simulink model "SOC_Estimation"  (R2020a)
settings: Solver=FixedStepDiscrete  StartTime=0.0  StopTime=10.0  FixedStep=0.05  RelTol=1e-3  EnableMultiTasking=on
InitFcn:
  | mbd_s32k_consistency_checks(bdroot(gcs));
values from neighbouring files (symbols this model uses):
  SOCInit = 0.75    [DD_SOC_Estimation.sldd]
  Ts = 0.1    [DD_SOC_Estimation.sldd]
undefined symbols (not defined in the file or in its folder): Battery, BMS_State_Enum, DiscIntNeverNeededParam, LQFP, Ns_Module, NumModules
libraries: simulink x6, sharedTrackingLibrary x2, mbd_s32k1xx_ec_toolbox x1
settings Model: DataDictionary=DD_SOC_Estimation.sldd  EnableAccessToBaseWorkspace=off  ExtModeTrigDuration=5  Creator=cpatel  LastModifiedBy=RolandoA
settings SolverCC: AutoInsertRateTranBlk=on
settings DataIOCC: ExternalInput=off  InitialState=off  SaveOutput=off  SignalLogging=off  SaveTime=off
settings OptimizationCC: DefaultParameterBehavior=Inlined  EnhancedBackFolding=on  PassReuseOutputArgsAs=Individual arguments  ZeroExternalMemoryAtStartup=off  ZeroInternalMemoryAtStartup=off  OptimizeBlockOrder=speed  DifferentSizesBufferReuse=on  OptimizationCustomize=off  EfficientTunableParamExpr=on
settings DebuggingCC: UnderspecifiedInitializationDetection=Classic  MergeDetectMultiDrivingBlocksExec=none  InheritedTsInSrcMsg=none  SingleTaskRateTransMsg=error  ParameterTunabilityLossMsg=error  UnconnectedInputMsg=error  UnconnectedOutputMsg=error  UnconnectedLineMsg=error  UnknownTsInhSupMsg=error
settings HardwareCC: ProdBitPerPointer=32  ProdBitPerSizeT=32  ProdBitPerPtrDiffT=32  ProdLargestAtomicInteger=Long  ProdLargestAtomicFloat=Double  ProdWordSize=32  ProdHWDeviceType=ARM Compatible->ARM Cortex
settings ModelReferenceCC: ModelReferenceNumInstancesAllowed=Single  PropagateSignalLabelsOutOfModel=off
settings SFSimCC: MATLABDynamicMemAlloc=off
settings RTWCC: Description=Model Based Design Toolbox S32K1xx Code Generation Target  SystemTargetFile=mbd_s32k.tlc  MakeCommand=mbd_s32k_make_rtw COPY_MDLREF_INCLUDES=0  TemplateMakefile=mbd_s32k.tmf  GenerateReport=on  IncludeHyperlinkInReport=on  LaunchReport=on  GenerateTraceInfo=on  GenerateTraceReport=on  GenerateTraceReportSl=on  GenerateTraceReportSf=on  GenerateTraceReportEml=on
settings CodeAppCC: ForceParamTrailComments=on  IgnoreCustomStorageClasses=off  OperatorAnnotations=on  SimulinkDataObjDesc=on  SFDataObjDesc=on  InsertBlockDesc=on
settings STFCustomTargetCC: TargetLangStandard=C99 (ISO)  MultiwordLength=256  CombineOutputUpdateFcns=on  ERTCustomFileBanners=on  SupportContinuousTime=off  SupportNonInlinedSFcns=off  RemoveResetFunc=on  MATLABClassNameForMDSCustomization=Simulink.SoftwareTarget.ERTCustomization  SystemTargetFile=mbd_s32k.tlc
settings ERTTargetCC: TargetLangStandard=C99 (ISO)  ParMdlRefBuildCompliant=off  CompOptLevelCompliant=off  ConcurrentExecutionCompliant=off  ModelStepFunctionPrototypeControlCompliant=off  CPPClassGenCompliant=off  UseToolchainInfoCompliant=off  InlinedParameterPlacement=NonHierarchical  ERTSrcFileBannerTemplate=mbd_ert_code_template.cgt  ERTHdrFileBannerTemplate=mbd_ert_code_template.cgt  ERTDataSrcFileTemplate=mbd_ert_code_template.cgt  ERTDataHdrFileTemplate=mbd_ert_code_template.cgt  ERTCustomFileTemplate=example_file_process.tlc

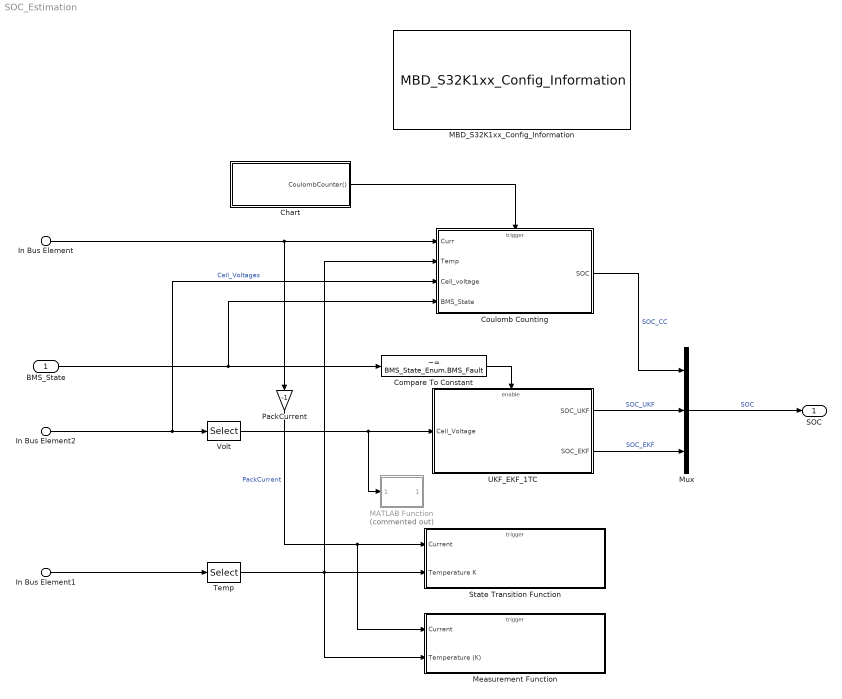
== system SOC_Estimation ==
  BMS_State : Inport  OutDataTypeStr=Enum: BMS_State_Enum
  In Bus Element2 : Inport  Port=2  PortName=BMS_Input  Element=Cell_Voltages
  In Bus Element : Inport  Port=2  PortName=BMS_Input  Element=Pack_Current
  In Bus Element1 : Inport  Port=2  PortName=BMS_Input  Element=Cell_Temperatures
  Chart : Stateflow chart  TreatAsAtomicUnit=on
  Compare To Constant : simulink/Logic and Bit Operations/Compare To Constant  relop=~=  const=BMS_State_Enum.BMS_Fault  OutDataTypeStr=boolean
  Coulomb Counting : Subsystem  VariantControl=SocAlgo==1
  MATLAB Function : MATLAB Function  Commented=on  TreatAsAtomicUnit=on
  MBD_S32K1xx_Config_Information : mbd_s32k1xx_ec_toolbox/MBD_S32K1xx_Config_Information  mbdt_ver=0  disp_str=|  config_params=[]  mcu_target_name=S32K144  mcu_target_package=100-LQFP  mcu_target_sram_size=64KB  mcu_system_clock_freq=80  mcu_xtal_freq=External 8  mcu_steptick_timer=LPIT Channel 0  mcu_steptick_prio=15  ds_import_enable=on  target_compiler=GCC  target_memory=FLASH  gcc_target_compile_opts=-mthumb -mfloat-abi=hard -mfpu=fpv4-sp-d16 -O1 -g -gstrict-dwarf  gcc_target_assemble_opts=-mthumb -mfloat-abi=hard -mfpu=fpv4-sp-d16 -g  gcc_target_link_opts=-mthumb -mfloat-abi=hard -mfpu=fpv4-sp-d16  gcc_target_default_lcf=on  gcc_target_user_lcf=S32K148_192_flash.ld  ghs_target_compile_opts=-cpu=cortexm4f -thumb -fpu=vfpv4_d16 -fsingle -Ogeneral -Wundef -Wimplicit-int -Wshadow -Wtrigraphs --no_commons --gnu_asm -gnu99 -gdwarf-2 -G  ghs_target_assemble_opts=-cpu=cortexm4f -fpu=vfpv4_d16  ghs_target_link_opts=-cpu=cortexm4f -thumb -fpu=vfpv4_d16  ghs_target_default_lcf=on  ghs_target_user_lcf=S32K148_192_flash.ld  iar_target_compile_opts=--cpu=Cortex-M4F --thumb --fpu=VFPv4_sp -Ol -e --debug --dlib_config normal  iar_target_assemble_opts=--cpu Cortex-M4F --thumb --fpu VFPv4_sp  iar_target_link_opts=--no_exceptions --vfe --inline  iar_target_default_lcf=on  iar_target_user_lcf=S32K148_192_flash.icf  pil_download_enable=off  rbl_download_enable=on  rbl_start_delay=5000  rbl_download_interface=OpenSDA  rbl_restart_request=off  rbl_com_port=Custom  rbl_com_port_custom=COM1  pil_download_rate=57600  pil_opensda_drive=Custom  pil_opensda_drive_custom=D  pil_uart_instance=1  pil_uart_rx=PTC6: [LPUART1_RX | Receive]  pil_uart_tx=PTC7: [LPUART1_TX | Transmit]  FTM_PWM_PcrCheckEnDis=on  FTM_Input_Edge_Inputs_PcrCheckEnDis=on  FTM_Dual_Edge_Inputs_PcrCheckEnDis=on  FTM_Quadrature_Inputs_PcrCheckEnDis=on  FTM_Hall_Sensor_Inputs_PcrCheckEnDis=on  LPTMR_PcrCheckEnDis=on  PIT_PcrCheckEnDis=on  RTC_PcrCheckEnDis=on  FlexCAN_PcrCheckEnDis=on  LIN_PcrCheckEnDis=on  FlexIO_PcrCheckEnDis=on  LPI2C_PcrCheckEnDis=on  LPSPI_PcrCheckEnDis=on  LPUART_PcrCheckEnDis=on  CMP_PcrCheckEnDis=on  GPIO_OutputPcrCheckEnDis=on  GPIO_InputPcrCheckEnDis=on  SBC_PcrCheckEnDis=on  BMS_PcrCheckEnDis=on  AMMCLIB_PcrCheckEnDis=on  FM_PcrCheckEnDis=on  Profile_PcrCheckEnDis=on  ConfigParams_PcrCheckEnDis=on  ModelRef_PcrCheckEnDis=on  PDB0_PcrCheckEnDis=on  CSEc_PcrCheckEnDis=on  eDMA_PcrCheckEnDis=on  FLASH_PcrCheckEnDis=on  ADC_PcrCheckEnDis=on  WDOG_PcrCheckEnDis=on
      | Target : S32K144-64KB_SRAM
      | Package : 100-pin
      | System clock : 80 MHz
      | XTAL clock : External 8 MHz
      | Compiler : IAR
      | Target Type : FLASH
      | Download Code after build : off
      | Step Tick Interrupt Priority : 15
  Measurement Function : Subsystem  TreatAsAtomicUnit=on
  Mux : Mux  Inputs=3
  PackCurrent : Gain  Gain=-1
  State Transition Function : Subsystem  TreatAsAtomicUnit=on
  Temp : Selector  InputPortWidth=Ns_Module*NumModules - 6  IndexOptions=Index vector (dialog)  Indices=[1]  OutputSizes=1
  UKF_EKF_1TC : Subsystem  VariantControl=CellType==1
  Volt : Selector  InputPortWidth=Ns_Module*NumModules  IndexOptions=Index vector (dialog)  Indices=[1]  OutputSizes=1
  SOC : Outport  OutDataTypeStr=single  VectorParamsAs1DForOutWhenUnconnected=off
  wires:
  In Bus Element2/1 -> Coulomb Counting/3(Cell_voltage), Volt/1  "Cell_Voltages"
  In Bus Element1/1 -> Temp/1
  Mux/1 -> SOC/1  "SOC"
  In Bus Element/1 -> Coulomb Counting/1(Curr), PackCurrent/1
  BMS_State/1 -> Coulomb Counting/4(BMS_State), Compare To Constant/1
  Compare To Constant/1 -> UKF_EKF_1TC/Enable
  PackCurrent/1 -> State Transition Function/1(Current), Measurement Function/1(Current)  "PackCurrent"
  Temp/1 -> Measurement Function/2(Temperature (K)), Coulomb Counting/2(Temp), State Transition Function/2(Temperature K)
  Volt/1 -> UKF_EKF_1TC/1(Cell_Voltage), MATLAB Function/1(meas)
  UKF_EKF_1TC/2(SOC_EKF) -> Mux/3  "SOC_EKF"
  UKF_EKF_1TC/1(SOC_UKF) -> Mux/2  "SOC_UKF"
  Chart/1(CoulombCounter()) -> Coulomb Counting/Trigger
  Coulomb Counting/1(SOC) -> Mux/1  "SOC_CC"

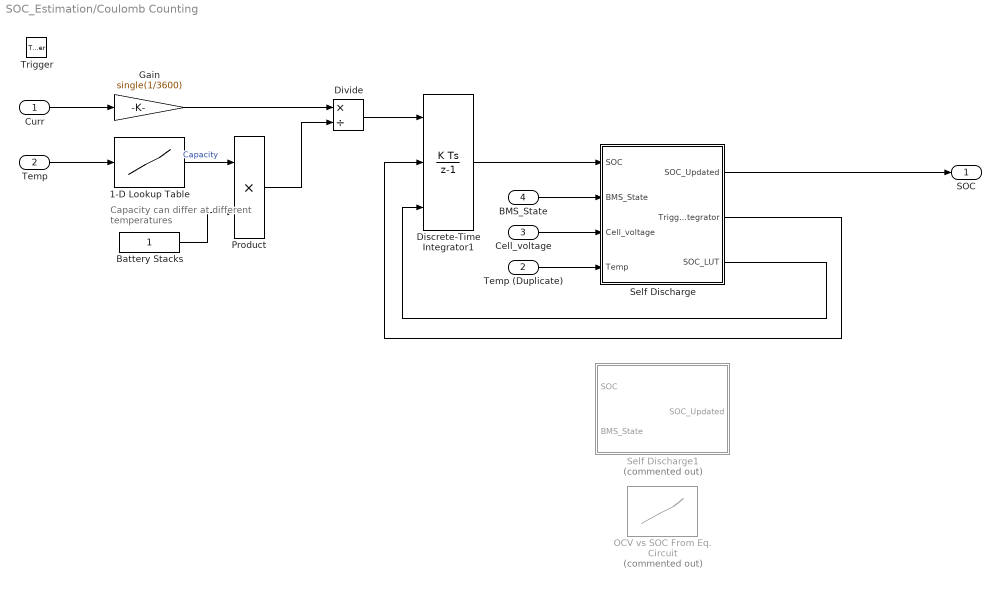
== system SOC_Estimation/Coulomb Counting ==
  note: Capacity can differ at different temperatures
  Curr : Inport
  Temp : Inport  Port=2
  Cell_voltage : Inport  Port=3
  BMS_State : Inport  Port=4
  Trigger : TriggerPort  TriggerType=function-call  VariantControl=Variant  PortDimensions=1
  1-D Lookup Table : Lookup_n-D  NumberOfTableDimensions=1  BreakpointsForDimension1=single(Battery.Temperature_LUT)  Table=single(Battery.Capacity_LUT)  InternalRulePriority=Speed  RndMeth=Simplest  InputSameDT=on
  Battery Stacks : Constant  OutDataTypeStr=single
  Discrete-Time Integrator1 : DiscreteIntegrator  ExternalReset=rising  InitialConditionSource=external  InitialCondition=single(SOCInit+0.05)  SampleTime=-1  LimitOutput=on  UpperSaturationLimit=1  LowerSaturationLimit=0  ICPrevOutput=DiscIntNeverNeededParam  ICPrevScaledInput=DiscIntNeverNeededParam
  Divide : Product  Inputs=*/
  Gain : Gain  Gain=single(1/3600)
  OCV vs SOC From Eq. Circuit : Lookup_n-D  Commented=on  NumberOfTableDimensions=1  BreakpointsForDimension1=single(Battery.Em_LUT1D)  Table=single(Battery.SOC_LUT)  InternalRulePriority=Speed  RndMeth=Simplest  InputSameDT=on
  Product : Product
  Self Discharge : Subsystem
  Self Discharge1 : Subsystem  Commented=on
  Temp (Duplicate) : InportShadow  Port=2
  SOC : Outport  VectorParamsAs1DForOutWhenUnconnected=off
  wires:
  Curr/1 -> Gain/1
  Gain/1 -> Divide/1
  Temp/1 -> 1-D Lookup Table/1
  1-D Lookup Table/1 -> Product/1  "Capacity"
  Product/1 -> Divide/2
  Battery Stacks/1 -> Product/2
  Self Discharge/1(SOC_Updated) -> SOC/1
  Self Discharge/2(Trigger_integrator) -> Discrete-Time Integrator1/2
  Self Discharge/3(SOC_LUT) -> Discrete-Time Integrator1/3
  Discrete-Time Integrator1/1 -> Self Discharge/1(SOC)
  Divide/1 -> Discrete-Time Integrator1/1
  BMS_State/1 -> Self Discharge/2(BMS_State)
  Cell_voltage/1 -> Self Discharge/3(Cell_voltage)
  Temp (Duplicate)/1 -> Self Discharge/4(Temp)

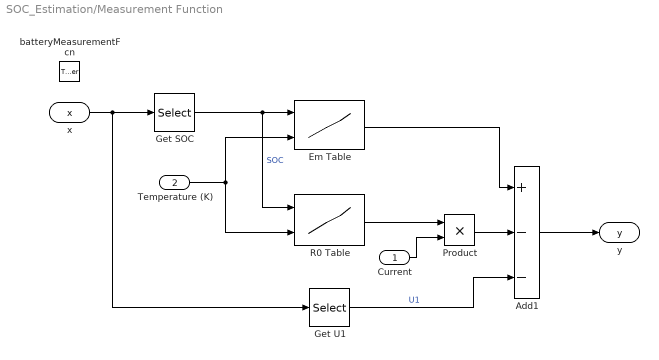
== system SOC_Estimation/Measurement Function ==
  Current : Inport
  Temperature (K) : Inport  Port=2
  batteryMeasurementFcn : TriggerPort  TriggerType=function-call  IsSimulinkFunction=on  FunctionName=batteryMeasurementFcn  VariantControl=Variant
  Add1 : Sum  Inputs=+--
  Em Table : Lookup_n-D  BreakpointsForDimension1=Battery.SOC_LUT  BreakpointsForDimension2=Battery.Temperature_LUT  BeginIndexSearchUsingPreviousIndexResult=on  Table=Battery.Em_LUT  ExtrapMethod=Clip  InternalRulePriority=Speed  RndMeth=Simplest  InputSameDT=on
  Get SOC : Selector  InputPortWidth=2  IndexOptions=Index vector (dialog)  Indices=[1]  OutputSizes=1
  Get U1 : Selector  InputPortWidth=2  IndexOptions=Index vector (dialog)  Indices=2  OutputSizes=1
  Product : Product
  R0 Table : Lookup_n-D  BreakpointsForDimension1=Battery.SOC_LUT  BreakpointsForDimension2=Battery.Temperature_LUT  BeginIndexSearchUsingPreviousIndexResult=on  Table=Battery.R0_LUT  ExtrapMethod=Clip  InternalRulePriority=Speed  RndMeth=Simplest  InputSameDT=on
  x : ArgIn  DisableCoverage=on  OutDataTypeStr=single  PortDimensions=2  ArgumentName=x
  y : ArgOut  DisableCoverage=on  OutDataTypeStr=single  ArgumentName=y
  wires:
  Get U1/1 -> Add1/3  "U1"
  Product/1 -> Add1/2
  Current/1 -> Product/2
  R0 Table/1 -> Product/1
  Temperature (K)/1 -> Em Table/2, R0 Table/2
  Add1/1 -> y/1
  Em Table/1 -> Add1/1
  Get SOC/1 -> Em Table/1, R0 Table/1  "SOC"
  x/1 -> Get SOC/1, Get U1/1

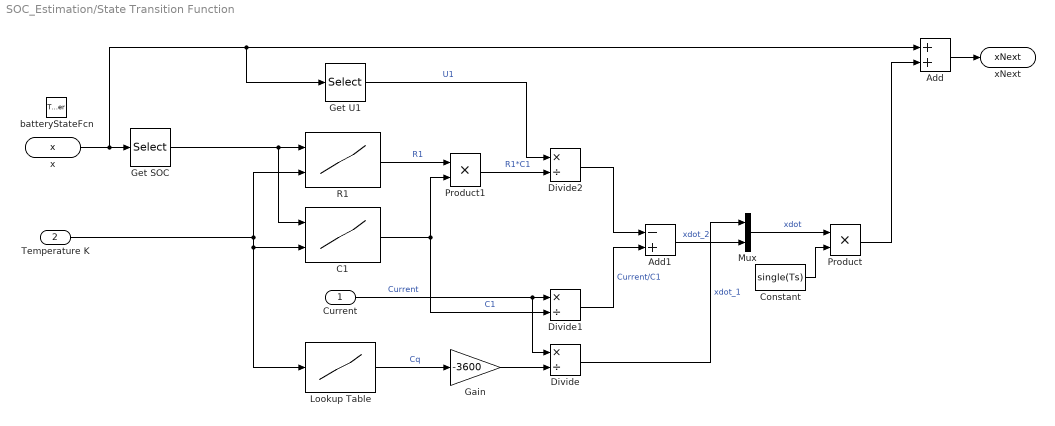
== system SOC_Estimation/State Transition Function ==
  Current : Inport
  Temperature K : Inport  Port=2
  batteryStateFcn : TriggerPort  TriggerType=function-call  IsSimulinkFunction=on  FunctionName=batteryStateFcn  VariantControl=Variant
  Add : Sum
  Add1 : Sum  Inputs=-+
  C1 : Lookup_n-D  BreakpointsForDimension1=Battery.SOC_LUT  BreakpointsForDimension2=Battery.Temperature_LUT  BeginIndexSearchUsingPreviousIndexResult=on  Table=Battery.C1_LUT  ExtrapMethod=Clip  InternalRulePriority=Speed  RndMeth=Simplest  InputSameDT=on
  Constant : Constant  Value=single(Ts)  OutDataTypeStr=single
  Divide : Product  Inputs=*/
  Divide1 : Product  Inputs=*/
  Divide2 : Product  Inputs=*/
  Gain : Gain  Gain=-3600
  Get SOC : Selector  InputPortWidth=2  IndexOptions=Index vector (dialog)  Indices=1  OutputSizes=1
  Get U1 : Selector  InputPortWidth=2  IndexOptions=Index vector (dialog)  Indices=2  OutputSizes=1
  Lookup Table : Lookup_n-D  NumberOfTableDimensions=1  BreakpointsForDimension1=Battery.Temperature_LUT  BeginIndexSearchUsingPreviousIndexResult=on  Table=Battery.Capacity_LUT  InternalRulePriority=Speed  RndMeth=Simplest  InputSameDT=on
  Mux : Mux  Inputs=2
  Product : Product  OutDataTypeStr=single
  Product1 : Product
  R1 : Lookup_n-D  BreakpointsForDimension1=Battery.SOC_LUT  BreakpointsForDimension2=Battery.Temperature_LUT  BeginIndexSearchUsingPreviousIndexResult=on  Table=Battery.R1_LUT  ExtrapMethod=Clip  InternalRulePriority=Speed  RndMeth=Simplest  InputSameDT=on
  x : ArgIn  DisableCoverage=on  OutDataTypeStr=single  PortDimensions=2  ArgumentName=x
  xNext : ArgOut  DisableCoverage=on  OutDataTypeStr=single  PortDimensions=2  ArgumentName=xNext
  wires:
  Lookup Table/1 -> Gain/1  "Cq"
  Product/1 -> Add/2
  Constant/1 -> Product/2
  Current/1 -> Divide1/1, Divide/1  "Current"
  Get SOC/1 -> C1/1, R1/1
  Temperature K/1 -> Lookup Table/1, C1/2, R1/2
  Add/1 -> xNext/1
  x/1 -> Add/1, Get U1/1, Get SOC/1
  Gain/1 -> Divide/2
  Divide/1 -> Mux/1  "xdot_1"
  Get U1/1 -> Divide2/1  "U1"
  Product1/1 -> Divide2/2  "R1*C1"
  R1/1 -> Product1/1  "R1"
  C1/1 -> Product1/2, Divide1/2  "C1"
  Divide1/1 -> Add1/2  "Current/C1"
  Divide2/1 -> Add1/1
  Add1/1 -> Mux/2  "xdot_2"
  Mux/1 -> Product/1  "xdot"

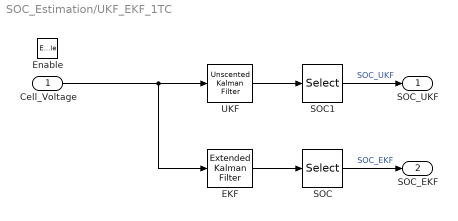
== system SOC_Estimation/UKF_EKF_1TC ==
  Cell_Voltage : Inport
  Enable : EnablePort
  EKF : sharedTrackingLibrary/Extended Kalman Filter  StateTransitionFcn=batteryStateFcn  HasStateTransitionJacobianFcn=off  HasAdditiveProcessNoise=Additive  ProcessNoise=1e-10*eye(2)  HasTimeVaryingProcessNoise=off  HasStateTransitionFcnExtraArgument=0  InitialState=[single(SOCInit+0.05); 0;]  InitialStateCovariance=[1e-5 1]  MeasurementFcn1=batteryMeasurementFcn  HasMeasurementJacobianFcn1=off  HasMeasurementEnablePort1=off  HasAdditiveMeasurementNoise1=Additive  MeasurementNoise1=1e-1  HasTimeVaryingMeasurementNoise1=off  HasMeasurementFcnExtraArgument1=0  MeasurementFcn2=myMeasurementFcn  HasMeasurementJacobianFcn2=off  HasMeasurementEnablePort2=off  HasAdditiveMeasurementNoise2=Additive  MeasurementNoise2=1  HasTimeVaryingMeasurementNoise2=off  HasMeasurementFcnExtraArgument2=0  MeasurementFcn3=myMeasurementFcn  HasMeasurementJacobianFcn3=off  HasMeasurementEnablePort3=off  HasAdditiveMeasurementNoise3=Additive  MeasurementNoise3=1  HasTimeVaryingMeasurementNoise3=off  HasMeasurementFcnExtraArgument3=0  MeasurementFcn4=myMeasurementFcn  HasMeasurementJacobianFcn4=off  HasMeasurementEnablePort4=off  HasAdditiveMeasurementNoise4=Additive  MeasurementNoise4=1  HasTimeVaryingMeasurementNoise4=off  HasMeasurementFcnExtraArgument4=0  MeasurementFcn5=myMeasurementFcn  HasMeasurementJacobianFcn5=off  HasMeasurementEnablePort5=off  HasAdditiveMeasurementNoise5=Additive  MeasurementNoise5=1  HasTimeVaryingMeasurementNoise5=off  HasMeasurementFcnExtraArgument5=0  EnableMultirate=off  StateTransitionFcnSampleTime=1  MeasurementFcn1SampleTime=1  MeasurementFcn2SampleTime=1  MeasurementFcn3SampleTime=1  MeasurementFcn4SampleTime=1  MeasurementFcn5SampleTime=1  UseCurrentEstimator=on  OutputStateCovariance=off  DataType=single  SampleTime=Ts  NumberOfMeasurements=1
      settings: SourceProductBaseCode=CT,DR,TF,ID,NV,AR,RO,VE
  SOC : Selector  InputPortWidth=2  IndexOptions=Index vector (dialog)  Indices=1  OutputSizes=1
  SOC1 : Selector  InputPortWidth=2  IndexOptions=Index vector (dialog)  Indices=1  OutputSizes=1
  UKF : sharedTrackingLibrary/Unscented Kalman Filter  StateTransitionFcn=batteryStateFcn  HasAdditiveProcessNoise=Additive  ProcessNoise=1e-10*eye(2)  HasTimeVaryingProcessNoise=off  HasStateTransitionFcnExtraArgument=0  InitialState=[single(SOCInit+0.05); 0;]  InitialStateCovariance=[1e-5 1]  Alpha=1  Beta=2  Kappa=1  MeasurementFcn1=batteryMeasurementFcn  HasMeasurementEnablePort1=off  HasAdditiveMeasurementNoise1=Additive  MeasurementNoise1=0.1  HasTimeVaryingMeasurementNoise1=off  HasMeasurementFcnExtraArgument1=0  MeasurementFcn2=myMeasurementFcn  HasMeasurementEnablePort2=off  HasAdditiveMeasurementNoise2=Additive  MeasurementNoise2=1  HasTimeVaryingMeasurementNoise2=off  HasMeasurementFcnExtraArgument2=0  MeasurementFcn3=myMeasurementFcn  HasMeasurementEnablePort3=off  HasAdditiveMeasurementNoise3=Additive  MeasurementNoise3=1  HasTimeVaryingMeasurementNoise3=off  HasMeasurementFcnExtraArgument3=0  MeasurementFcn4=myMeasurementFcn  HasMeasurementEnablePort4=off  HasAdditiveMeasurementNoise4=Additive  MeasurementNoise4=1  HasTimeVaryingMeasurementNoise4=off  HasMeasurementFcnExtraArgument4=0  MeasurementFcn5=myMeasurementFcn  HasMeasurementEnablePort5=off  HasAdditiveMeasurementNoise5=Additive  MeasurementNoise5=1  HasTimeVaryingMeasurementNoise5=off  HasMeasurementFcnExtraArgument5=0  EnableMultirate=off  StateTransitionFcnSampleTime=-1  MeasurementFcn1SampleTime=-1  MeasurementFcn2SampleTime=-1  MeasurementFcn3SampleTime=-1  MeasurementFcn4SampleTime=-1  MeasurementFcn5SampleTime=-1  UseCurrentEstimator=on  OutputStateCovariance=off  DataType=single  SampleTime=Ts  NumberOfMeasurements=1
      settings: SourceProductBaseCode=CT,DR,TF,ID,NV,AR,RO,VE
  SOC_UKF : Outport  VectorParamsAs1DForOutWhenUnconnected=off
  SOC_EKF : Outport  Port=2  VectorParamsAs1DForOutWhenUnconnected=off
  wires:
  UKF/1 -> SOC1/1
  Cell_Voltage/1 -> UKF/1, EKF/1
  SOC1/1 -> SOC_UKF/1  "SOC_UKF"
  EKF/1 -> SOC/1
  SOC/1 -> SOC_EKF/1  "SOC_EKF"

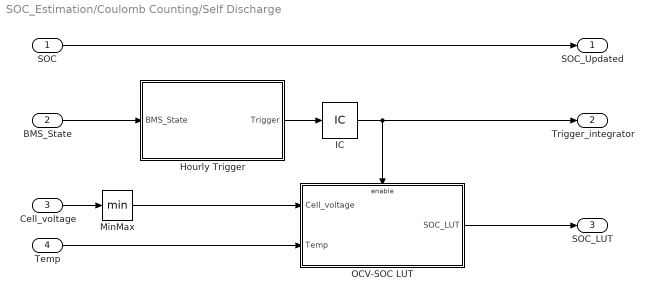
== system SOC_Estimation/Coulomb Counting/Self Discharge ==
  SOC : Inport
  BMS_State : Inport  Port=2
  Cell_voltage : Inport  Port=3
  Temp : Inport  Port=4
  Hourly Trigger : Subsystem
  IC : InitialCondition
  MinMax : MinMax
  OCV-SOC LUT : Subsystem
  SOC_Updated : Outport
  Trigger_integrator : Outport  Port=2
  SOC_LUT : Outport  Port=3
  wires:
  Hourly Trigger/1(Trigger) -> IC/1
  BMS_State/1 -> Hourly Trigger/1(BMS_State)
  SOC/1 -> SOC_Updated/1
  Cell_voltage/1 -> MinMax/1
  OCV-SOC LUT/1(SOC_LUT) -> SOC_LUT/1
  IC/1 -> Trigger_integrator/1, OCV-SOC LUT/Enable
  MinMax/1 -> OCV-SOC LUT/1(Cell_voltage)
  Temp/1 -> OCV-SOC LUT/2(Temp)

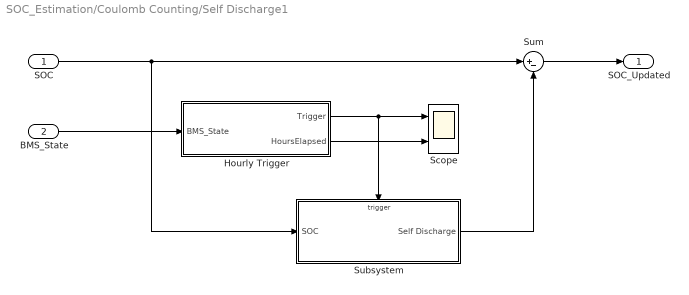
== system SOC_Estimation/Coulomb Counting/Self Discharge1 ==
  SOC : Inport
  BMS_State : Inport  Port=2
  Hourly Trigger : Subsystem
  Scope : Scope  NumInputPorts=2
  Subsystem : Subsystem
  Sum : Sum  Inputs=|+-
  SOC_Updated : Outport
  wires:
  SOC/1 -> Subsystem/1(SOC), Sum/1
  Sum/1 -> SOC_Updated/1
  Subsystem/1(Self Discharge) -> Sum/2
  BMS_State/1 -> Hourly Trigger/1(BMS_State)
  Hourly Trigger/1(Trigger) -> Scope/1, Subsystem/Trigger
  Hourly Trigger/2(HoursElapsed) -> Scope/2

== system SOC_Estimation/Coulomb Counting/Self Discharge/Hourly Trigger ==
  BMS_State : Inport
  1hr Trigger : Subsystem
  Compare To Constant1 : simulink/Logic and Bit Operations/Compare To Constant  relop===  const=BMS_State_Enum.BMS_Standby  OutDataTypeStr=boolean
  Trigger : Outport
  wires:
  BMS_State/1 -> Compare To Constant1/1
  Compare To Constant1/1 -> 1hr Trigger/Enable
  1hr Trigger/1(Trigger) -> Trigger/1

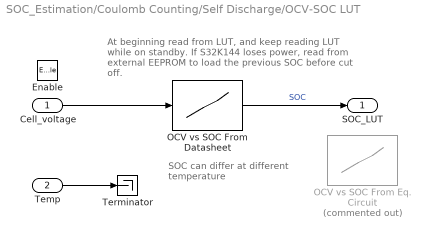
== system SOC_Estimation/Coulomb Counting/Self Discharge/OCV-SOC LUT ==
  note: SOC can differ at different temperature
  note: At beginning read from LUT, and keep reading LUT while on standby. If S32K144 loses power, read from external EEPROM to load the previous SOC before cut off.
  Cell_voltage : Inport
  Temp : Inport  Port=2
  Enable : EnablePort
  OCV vs SOC From Datasheet : Lookup_n-D  NumberOfTableDimensions=1  BreakpointsForDimension1=single(Battery.OCVLUT_DS)  Table=single(Battery.SOCLUT_DS)  InternalRulePriority=Speed  RndMeth=Simplest  InputSameDT=on
  OCV vs SOC From Eq. Circuit : Lookup_n-D  Commented=on  NumberOfTableDimensions=1  BreakpointsForDimension1=single(Battery.Em_LUT1D)  Table=single(Battery.SOC_LUT)  InternalRulePriority=Speed  RndMeth=Simplest  InputSameDT=on
  Terminator : Terminator
  SOC_LUT : Outport
  wires:
  OCV vs SOC From Datasheet/1 -> SOC_LUT/1  "SOC"
  Cell_voltage/1 -> OCV vs SOC From Datasheet/1
  Temp/1 -> Terminator/1

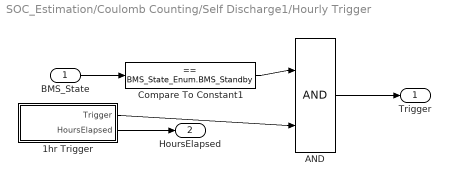
== system SOC_Estimation/Coulomb Counting/Self Discharge1/Hourly Trigger ==
  BMS_State : Inport
  1hr Trigger : Subsystem
  AND : Logic  IconShape=distinctive  AllPortsSameDT=off  OutDataTypeStr=boolean
  Compare To Constant1 : simulink/Logic and Bit Operations/Compare To Constant  relop===  const=BMS_State_Enum.BMS_Standby  OutDataTypeStr=boolean
  Trigger : Outport
  HoursElapsed : Outport  Port=2
  wires:
  BMS_State/1 -> Compare To Constant1/1
  AND/1 -> Trigger/1
  1hr Trigger/1(Trigger) -> AND/2
  1hr Trigger/2(HoursElapsed) -> HoursElapsed/1
  Compare To Constant1/1 -> AND/1

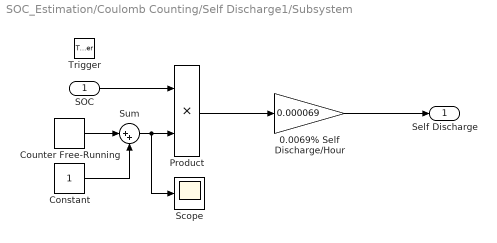
== system SOC_Estimation/Coulomb Counting/Self Discharge1/Subsystem ==
  SOC : Inport
  Trigger : TriggerPort  VariantControl=Variant  PortDimensions=1
  0.0069% Self Discharge/Hour : Gain  Gain=0.000069
  Constant : Constant
  Counter Free-Running : simulink/Sources/Counter Free-Running  NumBits=64  tsamp=-1
  Product : Product
  Scope : Scope
  Sum : Sum  Inputs=|++
  Self Discharge : Outport
  wires:
  Product/1 -> 0.0069% Self Discharge/Hour/1
  0.0069% Self Discharge/Hour/1 -> Self Discharge/1
  SOC/1 -> Product/1
  Sum/1 -> Scope/1, Product/2
  Counter Free-Running/1 -> Sum/1
  Constant/1 -> Sum/2

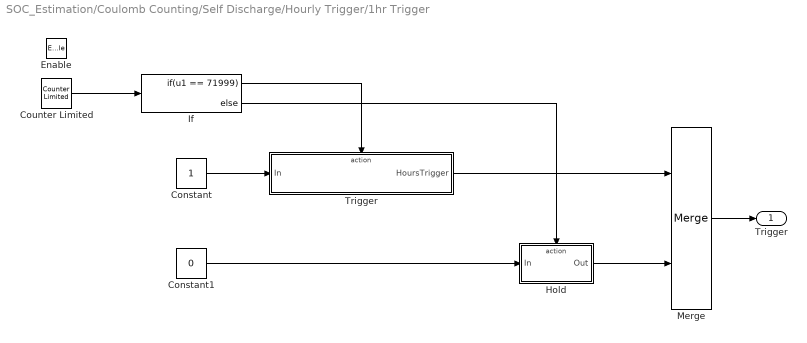
== system SOC_Estimation/Coulomb Counting/Self Discharge/Hourly Trigger/1hr Trigger ==
  Enable : EnablePort  StatesWhenEnabling=reset
  " Trigger" : Subsystem  TreatAsAtomicUnit=on
  Constant : Constant  OutDataTypeStr=uint16
  Constant1 : Constant  Value=0  OutDataTypeStr=uint16
  Counter Limited : simulink/Sources/Counter Limited  uplimit=71999  tsamp=-1
  Hold : Subsystem  TreatAsAtomicUnit=on
  If : If  IfExpression=u1 == 71999
  Merge : Merge
  Trigger : Outport  OutputWhenDisabled=reset  InitialOutput=0
  wires:
  " Trigger"/1(HoursTrigger) -> Merge/1
  If/1 -> " Trigger"/Action
  If/2 -> Hold/Action
  Merge/1 -> Trigger/1
  Constant1/1 -> Hold/1(In)
  Counter Limited/1 -> If/1
  Hold/1(Out) -> Merge/2
  Constant/1 -> " Trigger"/1(In)

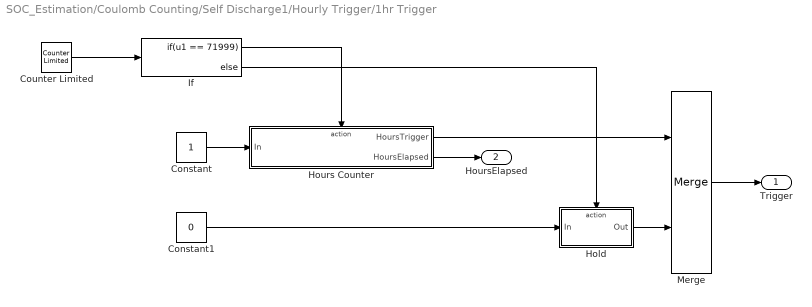
== system SOC_Estimation/Coulomb Counting/Self Discharge1/Hourly Trigger/1hr Trigger ==
  Constant : Constant  OutDataTypeStr=uint16
  Constant1 : Constant  Value=0  OutDataTypeStr=uint16
  Counter Limited : simulink/Sources/Counter Limited  uplimit=71999  tsamp=-1
  Hold : Subsystem  TreatAsAtomicUnit=on
  Hours Counter : Subsystem  TreatAsAtomicUnit=on
  If : If  IfExpression=u1 == 71999
  Merge : Merge
  Trigger : Outport
  HoursElapsed : Outport  Port=2
  wires:
  Constant/1 -> Hours Counter/1(In)
  Hold/1(Out) -> Merge/2
  Counter Limited/1 -> If/1
  Constant1/1 -> Hold/1(In)
  Merge/1 -> Trigger/1
  If/2 -> Hold/Action
  If/1 -> Hours Counter/Action
  Hours Counter/2(HoursElapsed) -> HoursElapsed/1
  Hours Counter/1(HoursTrigger) -> Merge/1

== system SOC_Estimation/Coulomb Counting/Self Discharge/Hourly Trigger/1hr Trigger/ Trigger ==
  In : Inport
  Action Port : ActionPort  ActionPortLabel=if(u1 == 71999)
  HoursTrigger : Outport  InitialOutput=0
  wires:
  In/1 -> HoursTrigger/1

== system SOC_Estimation/Coulomb Counting/Self Discharge/Hourly Trigger/1hr Trigger/Hold ==
  In : Inport
  Action Port : ActionPort  ActionPortLabel=else
  Out : Outport
  wires:
  In/1 -> Out/1

== system SOC_Estimation/Coulomb Counting/Self Discharge1/Hourly Trigger/1hr Trigger/Hold ==
  In : Inport
  Action Port : ActionPort
  Out : Outport
  wires:
  In/1 -> Out/1

== system SOC_Estimation/Coulomb Counting/Self Discharge1/Hourly Trigger/1hr Trigger/Hours Counter ==
  In : Inport
  Action Port : ActionPort
  Sum : Sum  Inputs=|++
  Unit Delay : UnitDelay  SampleTime=-1  HasFrameUpgradeWarning=on
  HoursTrigger : Outport
  HoursElapsed : Outport  Port=2
  wires:
  In/1 -> HoursTrigger/1, Sum/1
  Unit Delay/1 -> Sum/2
  Sum/1 -> HoursElapsed/1, Unit Delay/1

== stateflow chart SOC_Estimation/Chart ==
  state Init
  state Call
    CoulombCounter;
  (default) -> Init
  Init -> Call : [after(1,sec)]
  events: CoulombCounter output FUNCTION_CALL_EVENT

== matlab function SOC_Estimation/MATLAB Function ==
  data: meas input double; xhatOut output double
function xhatOut  = EXTKALMAN(meas)
%EXTKALMAN Radar Data Processing Tracker Using an Extended Kalman Filter
%
%  This program is executed as a MATLAB function block in the 
%  sldemo_radar Simulink model.  The estimated and actual positions are 
%  saved to the workspace and are plotted at the end of the simulation by 
%  the program aero_radplot (called from the simulation automatically).
%
%

%  Copyright 1990-2013 The MathWorks, Inc.
deltat = 0.1;
% Initialization
persistent P;
persistent xhat
if isempty(P)
    xhat = [0.75; 0];
    P = 1e-10*eye(2);
end
    
%  Radar update time deltat is inherited from model workspace

% 1. Compute Phi, Q, and R 
Phi = [1 deltat; 0 1];
%Phi = deltat;
Q =  1e-10*eye(2);
R =  1e-1;

% 2. Propagate the covariance matrix:
P = Phi*P*Phi' + Q;

% 3. Propagate the track estimate::
xhat = Phi*xhat;

% 4 a). Compute observation estimates:
xNext = batteryStateFnc(xhat);

% 4 b). Compute observation vector y and linearized measurement matrix M 
yhat = batteryMeasurementFcn(xhat);
M = [ cos(xNext(1))          0 sin(xNext(1))          0
   -sin(xNext(1))/xNext(2) 0 cos(xNext(1))/xNext(2) 0 ];
% 4 c).  Compute residual (Estimation Error)
residual = meas - yhat;

% 5. Compute Kalman Gain:
W = P*M'*inv(M*P*M'+ R);

% 6. Update estimate
xhat = xhat + W*residual;

% 7. Update Covariance Matrix
P = (eye(4)-W*M)*P*(eye(4)-W*M)' + W*R*W';

xhatOut = xhat;
